simulink model "Robust_passivity"  (R2021a)
settings: Solver=VariableStepAuto  StartTime=0.0  StopTime=10  FixedStep=.001  MaxStep=.1  RelTol=1e-3
settings Model: Creator=imi  LastModifiedBy=061
settings SolverCC: AlgebraicLoopSolver=TrustRegion
settings DataIOCC: ReturnWorkspaceOutputs=off
settings DebuggingCC: SFMachineParentedDataDiag=warning  ArithmeticOperatorsInVariantConditions=warning
settings SFSimCC: SimUseLocalCustomCode=off  CustomCodeUndefinedFunction=UseInterfaceOnly
settings RTWCC: RTWUseLocalCustomCode=off
settings CodeAppCC: StateflowObjectComments=on

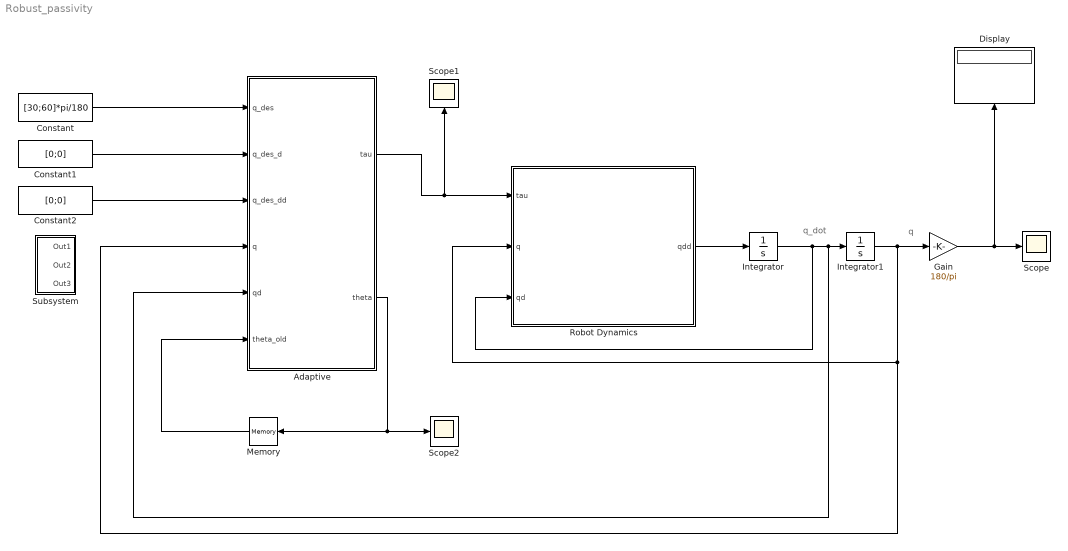
== system Robust_passivity ==
  note: q
  note: q_dot
  Adaptive : MATLAB Function  TreatAsAtomicUnit=on
  Constant : Constant  Value=[30;60]*pi/180
  Constant1 : Constant  Value=[0;0]
  Constant2 : Constant  Value=[0;0]
  Display : Display
  Gain : Gain  Gain=180/pi
  Integrator : Integrator  InitialCondition=zeros(2,1)
  Integrator1 : Integrator  InitialCondition=[45;95]*pi/180*0
  Memory : Memory  InitialCondition=rand(9,1)
  Robot Dynamics : MATLAB Function  TreatAsAtomicUnit=on
  Scope : Scope
  Scope1 : Scope
  Scope2 : Scope
  Subsystem : Subsystem
  wires:
  Integrator/1 -> Adaptive/5(qd), Integrator1/1, Robot Dynamics/3(qd)
  Integrator1/1 -> Adaptive/4(q), Robot Dynamics/2(q), Gain/1
  Gain/1 -> Scope/1, Display/1
  Constant/1 -> Adaptive/1(q_des)
  Constant1/1 -> Adaptive/2(q_des_d)
  Robot Dynamics/1(qdd) -> Integrator/1
  Adaptive/1(tau) -> Robot Dynamics/1(tau), Scope1/1
  Constant2/1 -> Adaptive/3(q_des_dd)
  Adaptive/2(theta) -> Memory/1, Scope2/1
  Memory/1 -> Adaptive/6(theta_old)

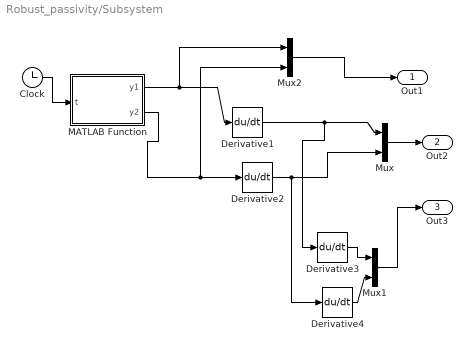
== system Robust_passivity/Subsystem ==
  Clock : Clock
  Derivative{1..4} (4 alike) : Derivative
  MATLAB Function : MATLAB Function  TreatAsAtomicUnit=on
  Mux : Mux  Inputs=2
  Mux1 : Mux  Inputs=2
  Mux2 : Mux  Inputs=2
  Out1 : Outport
  Out2 : Outport  Port=2
  Out3 : Outport  Port=3
  wires:
  Clock/1 -> MATLAB Function/1(t)
  Derivative2/1 -> Derivative4/1, Mux/2
  MATLAB Function/2(y2) -> Mux2/2, Derivative2/1
  Derivative1/1 -> Derivative3/1, Mux/1
  MATLAB Function/1(y1) -> Mux2/1, Derivative1/1
  Mux1/1 -> Out3/1
  Mux/1 -> Out2/1
  Derivative3/1 -> Mux1/1
  Derivative4/1 -> Mux1/2
  Mux2/1 -> Out1/1

== matlab function Robust_passivity/Robot Dynamics ==
  data: tau input; q input; qdd output; qd input
function qdd = fcn(tau,q,qd)

q1=q(1);
q2=q(2);

q1d=qd(1);
q2d=qd(2);



m1=2;
m2=1.4;

I1=.5;
I2=.1;

l1=.8;
l2=.8;

lc1=.4;
lc2=.4;


g=9.81;



d11=m1*lc1^2+I1+I2+m2*(l1^2+lc2^2+2*l1*lc2*cos(q2));
d12=m2*lc2^2+I2+m2*l2*lc2*cos(q2);
d21=m2*lc2^2+I2+m2*l2*lc2*cos(q2);
d22=m2*lc2^2+I2;

c11=-m2*l1*lc2*sin(q2)*q2d;
c12=-m2*l1*lc2*sin(q2)*(q1d+q2d);
c21=m2*l1*lc2*sin(q2)*q1d;
c22=0;

g11=m1*lc1*g*cos(q1)+m2*g*(lc2*cos(q1+q2)+l1*cos(q1));
g21=m2*lc2*g*cos(q1+q2);

M=[d11,d12;d21,d22];
C=[c11 c12;c21 c22];
G=[g11;g21];


qdd=pinv(M)*(tau-C*qd-G);

== matlab function Robust_passivity/Subsystem/MATLAB Function ==
  data: t input; y1 output; y2 output
function [y1,y2]= fcn(t)

y1=sin(.1*t);
y2=sin(.05*t+pi/6);

== matlab function Robust_passivity/Adaptive ==
  data: q_des input; q_des_d input; q_des_dd input; q input; qd input; tau output; theta output; theta_old input
function [tau,theta]= fcn(q_des,q_des_d,q_des_dd,q,qd,theta_old)

q1=q(1);
q2=q(2);

q1d=qd(1);
q2d=qd(2);




zita=1;
wn=2*pi*3;
K1=eye(2)*2*zita*wn;
K0=eye(2)*wn^2;

A=[zeros(2,2),eye(2);
    -K0,-K1];
B=[zeros(2,2);eye(2)];

P=[  0.0664         0   -0.5000         0;
    0    0.0664         0   -0.5000;
    -0.5000         0    4.7257         0;
    0   -0.5000         0    4.7257];

q_tilde=q-q_des;
q_tilde_d=qd-q_des_d;
e=[q_tilde;q_tilde_d];

q_tilde=q-q_des;
q_tilde_d=qd-q_des_d;

gamma=5;

q1=q(1);
q2=q(2);

q1d=qd(1);
q2d=qd(2);




v=q_des_d-gamma*q_tilde;
v_d=q_des_dd-gamma*q_tilde_d;
r=qd-v;

Y1=[v_d(1),v_d(2),v(1)*q2d+v(2)*q1d+q2d*v(2),cos(q1),cos(q1+q2)];
Y2=[v_d(1),v_d(2),q1d*v(1),cos(q1+q2)];
Y=blkdiag(Y1,Y2);

n=norm(Y'*r);
ee=2;
rho=5;
if(n>ee) 
    delta_theta=-rho*Y'*r/n;
else
    delta_theta=-rho*Y'*r/ee;
end

theta=theta_old+delta_theta;
K=11*eye(2);
tau=Y*theta-K*r;
